simulink model "Modello_attuatore"  (R2023a)
settings: Solver=ode14x  StartTime=0.0  StopTime=3  FixedStep=dt_sim  RelTol=1e-3
values from neighbouring files (symbols this model uses):
  A1_la = 5.710000e-003    (= 0.00571)    [C1_Actuator_1_Data.m]
  A2_la = 5.710000e-003    (= 0.00571)    [C1_Actuator_1_Data.m]
  a_jetpipe_area = 0    [B2_Main_file_Double_Active_Standby_System.m]
  A_svfb = 79.12.*1E-9.*sqrt(pi)    [B2_Main_file_Double_Active_Standby_System.m]
  a_svfb0_1 = 1E-3    (= 0.001)    [B2_Main_file_Double_Active_Standby_System.m]
  a_svfb0_2 = 0    [B2_Main_file_Double_Active_Standby_System.m]
  Afl_sv = dfl_sv^2*pi/4    (= 2.01519637574e-09)    [C1_Actuator_1_Data.m]
  Ag_sv = 18e-6    (= 1.8e-05)    [C1_Actuator_1_Data.m]
  air_gap0_1 = 0    [B2_Main_file_Double_Active_Standby_System.m]
  air_gap_fault_time = 10000    [B2_Main_file_Double_Active_Standby_System.m]
  Asp_sv = 1.35e-5    (= 1.35e-05)    [C1_Actuator_1_Data.m]
  B0_sv = 0.460    (= 0.46)    [C1_Actuator_1_Data.m]
  b_airgap = 0.3    [B2_Main_file_Double_Active_Standby_System.m]
  b_fbspring = 2E-3    (= 0.002)    [B2_Main_file_Double_Active_Standby_System.m]
  b_max = 0*0.0001    (= 0)    [C1_Actuator_1_Data.m]
  beta = 800000000    [D4_Fluid.m]    (also in Rapporto_di_trasmissione.m = acos((L-t.*cos(alpha))./s))
  beta_LVDT = 0    [aggiunte.m]
  bf_sv = 0.45    [C1_Actuator_1_Data.m]
  bsp_sv = 0.25    [C1_Actuator_1_Data.m]
  C_svfb = 1    [B2_Main_file_Double_Active_Standby_System.m]
  Cdmax_sv = 0.7392    [C1_Actuator_1_Data.m]
  Cdmin_sv = 0.6428    [C1_Actuator_1_Data.m]
  CLa = 900000    [aggiunte.m]
  Csa_la = 0.02*sqrt(Ksa_la*Meq_la)    [C1_Actuator_1_Data.m]
  Del_on = 1    [B2_Main_file_Double_Active_Standby_System.m]
  demag0_1 = 0    [B2_Main_file_Double_Active_Standby_System.m]
  dfl_sv = 5.0654e-5    (= 5.0654e-05)    [C1_Actuator_1_Data.m]
  dt_sim = 1e-5    (= 1e-05)    [B2_Main_file_Double_Active_Standby_System.m]
  enable_jetpipe_distorsion = 0    [B2_Main_file_Double_Active_Standby_System.m]
  F_att_sv = 4    [C1_Actuator_1_Data.m]
  FH = FH+0.175*pi*Dd_se(ii)*(-0.884+0.0206*Hs_se(ii)-0.0001*(Hs_se(ii))^2)*Tw_se(ii)    [D2_Data_seal.m]
  first_cycle = 0    [B2_Main_file_Double_Active_Standby_System.m]
  flight_hours = 8    [B2_Main_file_Double_Active_Standby_System.m]
  g_sv = G_sv/l0_sv    (= 0)    [C1_Actuator_1_Data.m]
  Gamma_la = 1.667e4    (= 16670)    [C1_Actuator_1_Data.m]
  gap_ms = 0    [C1_Actuator_1_Data.m]
  Gq_sv = 0.069    [C1_Actuator_1_Data.m]
  Gust_stiffness_jetpipe = 1e8    (= 100000000)    [B2_Main_file_Double_Active_Standby_System.m]
  Gust_threshold = 10000    [B2_Main_file_Double_Active_Standby_System.m]
  h_fbspring = 1E-3    (= 0.001)    [B2_Main_file_Double_Active_Standby_System.m]
  h_sv = H_sv/l0_sv    (= 0)    [C1_Actuator_1_Data.m]
  hr_sv = 6e-6    (= 6e-06)    [C1_Actuator_1_Data.m]
  hyd_fluid_repl = 20    [B2_Main_file_Double_Active_Standby_System.m]
  imax_sv = 8e-3    (= 0.008)    [C1_Actuator_1_Data.m]
  Ja_sv = 1.0575e-5    (= 1.0575e-05)    [C1_Actuator_1_Data.m]
  jetpipe_initialpos = 0    [B2_Main_file_Double_Active_Standby_System.m]
  jetpipe_passage_area = 1    [B2_Main_file_Double_Active_Standby_System.m]
  k_airgap = 0.5/100*0.01    (= 5e-05)    [B2_Main_file_Double_Active_Standby_System.m]
  k_c0_jetpipe_area = 0*1e-1    (= 0)    [B2_Main_file_Double_Active_Standby_System.m]
  k_sv = mup_sv*Vp_sv/(2*B0_sv*l0_sv)-1    (= 16.0383594613)    [C1_Actuator_1_Data.m]
  Kf_sv = 301.6    [C1_Actuator_1_Data.m]
  KFPi = zeros(m,1)    [D2_Data_seal.m]
  Kli1 = 0    [C1_Actuator_1_Data.m]
  Kli2 = 0    [C1_Actuator_1_Data.m]
  Ksa_la = 12480000    [C1_Actuator_1_Data.m]
  Kw_sv = 14.5    [C1_Actuator_1_Data.m]
  l0_sv = 0.5e-3    (= 0.0005)    [C1_Actuator_1_Data.m]
  L_c = imax_sv    (= 0.008)    [C1_Actuator_1_Data.m]
  L_la1 = 0.059900    (= 0.0599)    [C1_Actuator_1_Data.m]
  L_la2 = 0.084800    (= 0.0848)    [C1_Actuator_1_Data.m]
  la_sv = 41e-3    (= 0.041)    [C1_Actuator_1_Data.m]
  lambda_LVDT = 0*0.005*1.5    (= 0)    [aggiunte.m]
  lf = 0.025    [C1_Actuator_1_Data.m]    (also in C2_Actuator_2_Data.m)
  LVDTsize0 = 1    [aggiunte.m]
  m_thermal = 0    [B2_Main_file_Double_Active_Standby_System.m]
  Mcyl_la = 30.425550    (= 30.42555)    [C1_Actuator_1_Data.m]
  Mrod_la = 11.313490    (= 11.31349)    [C1_Actuator_1_Data.m]
  msp_sv = 0.005    [C1_Actuator_1_Data.m]
  mua_sv = 4*pi/1e7    (= 1.25663706144e-06)    [C1_Actuator_1_Data.m]
  mup_sv = 1.1*4*pi/1e7    (= 1.38230076758e-06)    [C1_Actuator_1_Data.m]
  n1_sv = 1140    [C1_Actuator_1_Data.m]
  n2_sv = 1140    [C1_Actuator_1_Data.m]
  n_svfb = 3    [B2_Main_file_Double_Active_Standby_System.m]
  null_shift = -1+2*rand(1,1)    [B2_Main_file_Double_Active_Standby_System.m]
  null_shift_sign = -1+((-1+2*rand(1,1))>=0)*2    [B2_Main_file_Double_Active_Standby_System.m]
  OV_R1 = 0*2.344e-05    (= 0)    [C1_Actuator_1_Data.m]
  OV_R2 = 0*2.344e-05    (= 0)    [C1_Actuator_1_Data.m]
  OV_S1 = 0*2.344e-05    (= 0)    [C1_Actuator_1_Data.m]
  OV_S2 = 0*2.344e-05    (= 0)    [C1_Actuator_1_Data.m]
  P01_la = Pmean-DP_eq    [C1_Actuator_1_Data.m]
  P02_la = Pmean+DP_eq    [C1_Actuator_1_Data.m]
  perc_passage_area0_1 = 0    [B2_Main_file_Double_Active_Standby_System.m]
  Pocl_A = 0    [C1_Actuator_1_Data.m]
  Pocl_B = 0    [C1_Actuator_1_Data.m]
  Pr = 600000    [B2_Main_file_Double_Active_Standby_System.m]
  Ps = 35000000    [B2_Main_file_Double_Active_Standby_System.m]
  R_th1 = 0    [B2_Main_file_Double_Active_Standby_System.m]
  Remax_sv = 5000    [C1_Actuator_1_Data.m]
  Resistance = 1    [C1_Actuator_1_Data.m]
  rj_sv = 1e-6    (= 1e-06)    [C1_Actuator_1_Data.m]
  Rp02_svspring = 1014    [B2_Main_file_Double_Active_Standby_System.m]
  sigma_0LVDT = 0*0.01*1.5*5    (= 0)    [aggiunte.m]
  ST_AD = ceil(10000/fs_AD)/10000    [C1_Actuator_1_Data.m]
  sv_crackON1 = 0    [B2_Main_file_Double_Active_Standby_System.m]
  sv_crackON2 = 0    [B2_Main_file_Double_Active_Standby_System.m]
  T0 = 0    [aggiunte.m]
  tau_w1 = 0    [B2_Main_file_Double_Active_Standby_System.m]
  Temperature_threshold = 0    [B2_Main_file_Double_Active_Standby_System.m]
  V01_la = (Vm_la1+A1_la*(L_la1+x0_la))    (= 0.00040017393)    [C1_Actuator_1_Data.m]
  V02_la = (Vm_la2+A2_la*(L_la2-x0_la))    (= 0.00056652336)    [C1_Actuator_1_Data.m]
  Voltage_com = Resistance    (= 1)    [C1_Actuator_1_Data.m]
  Vp_sv = 5.67e3    (= 5670)    [C1_Actuator_1_Data.m]
  w_fb = 310    [C1_Actuator_1_Data.m]
  w_sv = W_sv/l0_sv    (= 0)    [C1_Actuator_1_Data.m]
  wsp_sv = 0.009334348785340    (= 0.00933434878534)    [C1_Actuator_1_Data.m]
  x0_la = 0    [C1_Actuator_1_Data.m]
  xf_sv_max = 3.05e-5    (= 3.05e-05)    [C1_Actuator_1_Data.m]
  xmax_sb = 5.5e-3    (= 0.0055)    [C1_Actuator_1_Data.m]
  xspmax_sv = 0.001250    (= 0.00125)    [C1_Actuator_1_Data.m]
  z_fb = 0.5    [C1_Actuator_1_Data.m]
undefined symbols (not defined in the file or in its folder): magnitude, Newton, R_sp_C, Raphson
libraries: simulink x13
(part 3 of 3)

== system Modello_attuatore/Actuation System/Servovalve/Servovalve Dynamic/Spool  dynamic/Flow Force/Q_max evaluation and flow angle variation/Variation of flow angle Q2 ==
  In3 : Inport
  In1 : Inport  Port=2
  Constant4 : Constant  Value=0.5
  Flow less than 0.05 : Fcn  Expr=1-10*u(1)
  Product5 : Product  Inputs=*/  SaturateOnIntegerOverflow=on  OutDataTypeStr=Inherit: Same as first input
  Switch : Switch  Criteria=u2 > Threshold  Threshold=0.05  SaturateOnIntegerOverflow=off  InputSameDT=off
  cos(teta) : Outport
  wires:
  Switch/1 -> cos(teta)/1
  Constant4/1 -> Switch/1
  Product5/1 -> Flow less than 0.05/1, Switch/2
  In1/1 -> Product5/1
  In3/1 -> Product5/2
  Flow less than 0.05/1 -> Switch/3
